simulink model "lab2_model2"  (R2021b)
settings: Solver=FixedStepAuto  StartTime=0.0  StopTime=60  FixedStep=0.001  RelTol=1e-3
libraries: cstblocks x16, qube2servo x6
settings Model: Creator=12288  LastModifiedBy=12288

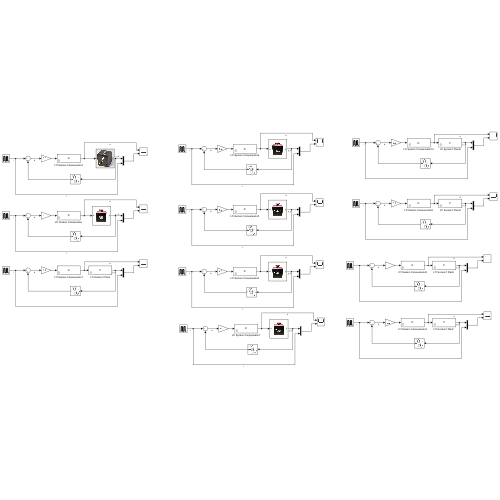
[thumbnail: Simulink's stored preview of the top-level diagram]
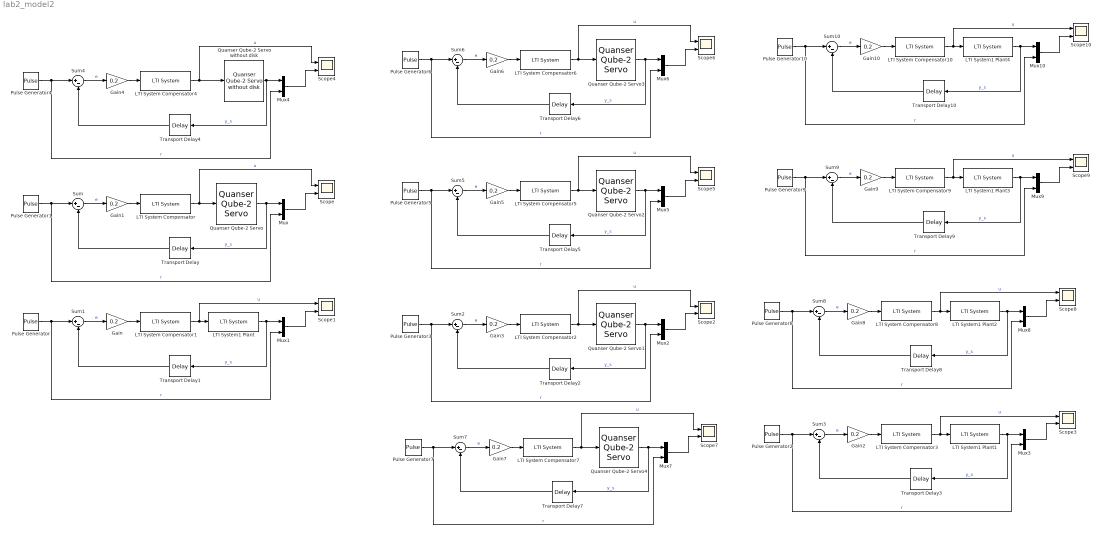
== system lab2_model2 ==
  Gain{,1..10} (11 alike) : Gain  Gain=0.2
  LTI System Compensator{,1..10} (11 alike) : cstblocks/LTI System  sys=D  IC=[]
  LTI System1 Plant{,1..4} (5 alike) : cstblocks/LTI System  sys=P  IC=[]
  Mux{,1..10} (11 alike) : Mux  Inputs=2
  Pulse Generator{,1..10} (11 alike) : DiscretePulseGenerator  PulseType=Time based  Period=10  PulseWidth=50
  Quanser Qube-2 Servo{,1..4} (5 alike) : qube2servo/Quanser Qube-2 Servo  SystemSampleTime=-1  VariantActivationTime=update diagram  Latency=0  AutoFrameSizeCalculation=off
  Quanser Qube-2 Servo without disk : qube2servo/Quanser Qube-2 Servo without disk  SystemSampleTime=-1  VariantActivationTime=update diagram  Latency=0  AutoFrameSizeCalculation=off
  Scope{,1..10} (11 alike) : Scope  NumInputPorts=2
  Sum{,1..10} (11 alike) : Sum  Inputs=|+-
  Transport Delay{,1,3..4,7} (5 alike) : TransportDelay  DelayTime=0
  Transport Delay10 : TransportDelay  DelayTime=0.45
  Transport Delay2 : TransportDelay  DelayTime=0.15
  Transport Delay5 : TransportDelay  DelayTime=0.3
  Transport Delay6 : TransportDelay  DelayTime=0.45
  Transport Delay8 : TransportDelay  DelayTime=0.15
  Transport Delay9 : TransportDelay  DelayTime=0.3
  wires:
  LTI System Compensator/1 -> Quanser Qube-2 Servo/1, Scope/1  "u"
  Quanser Qube-2 Servo/1 -> Mux/1, Transport Delay/1  "y_s"
  Pulse Generator1/1 -> Mux/2, Sum/1  "r"
  Sum/1 -> Gain1/1  "e"
  Transport Delay/1 -> Sum/2
  Gain1/1 -> LTI System Compensator/1
  Mux/1 -> Scope/2
  Sum1/1 -> Gain/1  "e"
  Transport Delay1/1 -> Sum1/2
  Mux1/1 -> Scope1/2
  LTI System1 Plant/1 -> Transport Delay1/1, Mux1/1  "y_s"
  Gain/1 -> LTI System Compensator1/1
  Pulse Generator/1 -> Mux1/2, Sum1/1  "r"
  LTI System Compensator1/1 -> Scope1/1, LTI System1 Plant/1  "u"
  Gain3/1 -> LTI System Compensator2/1
  Mux2/1 -> Scope2/2
  Pulse Generator3/1 -> Mux2/2, Sum2/1  "r"
  LTI System Compensator2/1 -> Quanser Qube-2 Servo1/1, Scope2/1  "u"
  Transport Delay2/1 -> Sum2/2
  Sum2/1 -> Gain3/1  "e"
  Quanser Qube-2 Servo1/1 -> Transport Delay2/1, Mux2/1  "y_s"
  Sum4/1 -> Gain4/1  "e"
  Transport Delay4/1 -> Sum4/2
  Gain4/1 -> LTI System Compensator4/1
  Mux4/1 -> Scope4/2
  Pulse Generator4/1 -> Mux4/2, Sum4/1  "r"
  Quanser Qube-2 Servo without disk/1 -> Transport Delay4/1, Mux4/1  "y_s"
  LTI System Compensator4/1 -> Quanser Qube-2 Servo without disk/1, Scope4/1  "u"
  Pulse Generator5/1 -> Mux5/2, Sum5/1  "r"
  Sum5/1 -> Gain5/1  "e"
  Quanser Qube-2 Servo2/1 -> Transport Delay5/1, Mux5/1  "y_s"
  Transport Delay5/1 -> Sum5/2
  LTI System Compensator5/1 -> Quanser Qube-2 Servo2/1, Scope5/1  "u"
  Mux5/1 -> Scope5/2
  Gain5/1 -> LTI System Compensator5/1
  Pulse Generator6/1 -> Mux6/2, Sum6/1  "r"
  Sum6/1 -> Gain6/1  "e"
  Quanser Qube-2 Servo3/1 -> Transport Delay6/1, Mux6/1  "y_s"
  Transport Delay6/1 -> Sum6/2
  LTI System Compensator6/1 -> Quanser Qube-2 Servo3/1, Scope6/1  "u"
  Mux6/1 -> Scope6/2
  Gain6/1 -> LTI System Compensator6/1
  Quanser Qube-2 Servo4/1 -> Transport Delay7/1, Mux7/1  "y_s"
  Sum7/1 -> Gain7/1  "e"
  Transport Delay7/1 -> Sum7/2
  LTI System Compensator7/1 -> Quanser Qube-2 Servo4/1, Scope7/1  "u"
  Gain7/1 -> LTI System Compensator7/1
  Pulse Generator7/1 -> Mux7/2, Sum7/1  "r"
  Mux7/1 -> Scope7/2
  Mux3/1 -> Scope3/2
  Gain2/1 -> LTI System Compensator3/1
  Transport Delay3/1 -> Sum3/2
  Pulse Generator2/1 -> Mux3/2, Sum3/1  "r"
  LTI System Compensator3/1 -> Scope3/1, LTI System1 Plant1/1  "u"
  LTI System1 Plant1/1 -> Transport Delay3/1, Mux3/1  "y_s"
  Sum3/1 -> Gain2/1  "e"
  Mux8/1 -> Scope8/2
  Gain8/1 -> LTI System Compensator8/1
  Transport Delay8/1 -> Sum8/2
  Pulse Generator8/1 -> Mux8/2, Sum8/1  "r"
  LTI System Compensator8/1 -> Scope8/1, LTI System1 Plant2/1  "u"
  LTI System1 Plant2/1 -> Transport Delay8/1, Mux8/1  "y_s"
  Sum8/1 -> Gain8/1  "e"
  Mux9/1 -> Scope9/2
  Gain9/1 -> LTI System Compensator9/1
  Transport Delay9/1 -> Sum9/2
  Pulse Generator9/1 -> Mux9/2, Sum9/1  "r"
  LTI System Compensator9/1 -> Scope9/1, LTI System1 Plant3/1  "u"
  LTI System1 Plant3/1 -> Transport Delay9/1, Mux9/1  "y_s"
  Sum9/1 -> Gain9/1  "e"
  Mux10/1 -> Scope10/2
  Gain10/1 -> LTI System Compensator10/1
  Transport Delay10/1 -> Sum10/2
  Pulse Generator10/1 -> Mux10/2, Sum10/1  "r"
  LTI System Compensator10/1 -> Scope10/1, LTI System1 Plant4/1  "u"
  LTI System1 Plant4/1 -> Transport Delay10/1, Mux10/1  "y_s"
  Sum10/1 -> Gain10/1  "e"
